simulink model "Test_sensor_drift"  (R2017b)
settings: Solver=VariableStepAuto  StartTime=0.0  StopTime=10.0  RelTol=1e-3
settings Model: Creator=dc0069  LastModifiedBy=dc0069

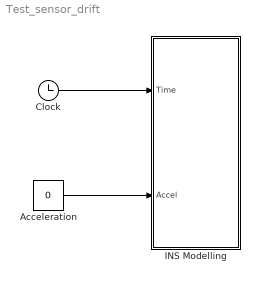
== system Test_sensor_drift ==
  Acceleration : Constant  Value=0
  Clock : Clock
  INS Modelling : Subsystem
  wires:
  Clock/1 -> INS Modelling/1(Time)
  Acceleration/1 -> INS Modelling/2(Accel)

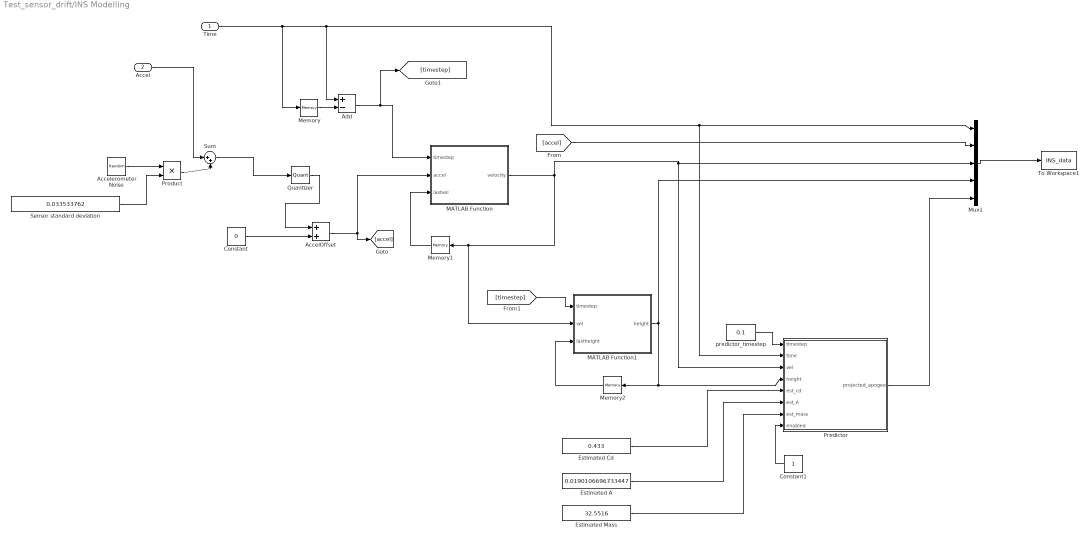
== system Test_sensor_drift/INS Modelling ==
  Time : Inport  SampleTime=.1
  Accel : Inport  Port=2  SampleTime=.1
  AccelOffset : Sum
  Accelerometer Noise : RandomNumber  Seed=3784  SampleTime=0.1  VectorParams1D=off
  Add : Sum  Inputs=+-
  Constant : Constant  Value=0
  Constant1 : Constant
  Estimated A : Constant  Value=0.0190106696733447
  Estimated Cd : Constant  Value=0.433
  Estimated Mass : Constant  Value=32.5516
  MATLAB Function : MATLAB Function  TreatAsAtomicUnit=on
  MATLAB Function1 : MATLAB Function  TreatAsAtomicUnit=on
  Memory : Memory
  Memory1 : Memory
  Memory2 : Memory
  Mux1 : Mux  Inputs=5
  Predictor : MATLAB Function  TreatAsAtomicUnit=on
  Product : Product
  Quantizer : Quantizer  QuantizationInterval=.01
  Sensor standard deviation : Constant  Value=0.033533762
  Sum : Sum  Inputs=|++
  To Workspace1 : ToWorkspace  VariableName=INS_data  SampleTime=.1
  "predictor_timestep " : Constant  Value=0.1
  wires:
  Accel/1 -> Sum/1
  Mux1/1 -> To Workspace1/1
  Time/1 -> Add/1, Predictor/2(time), Mux1/1, Memory/1
  AccelOffset/1 -> MATLAB Function/2(accel), [accel]
  Memory/1 -> Add/2
  Add/1 -> [timestep], MATLAB Function/1(timestep)
  [accel] -> Mux1/2
  MATLAB Function/1(velocity) -> MATLAB Function1/2(vel), Memory1/1, Mux1/3, Predictor/3(vel)
  Memory1/1 -> MATLAB Function/3(lastvel)
  Sum/1 -> Quantizer/1
  [timestep] -> MATLAB Function1/1(timestep)
  MATLAB Function1/1(height) -> Mux1/4, Predictor/4(height), Memory2/1
  Memory2/1 -> MATLAB Function1/3(lastheight)
  Predictor/1(projected_apogee) -> Mux1/5
  Quantizer/1 -> AccelOffset/1
  Constant/1 -> AccelOffset/2
  Estimated Cd/1 -> Predictor/5(est_cd)
  Estimated A/1 -> Predictor/6(est_A)
  Estimated Mass/1 -> Predictor/7(est_mass)
  "predictor_timestep "/1 -> Predictor/1(timestep)
  Sensor standard deviation/1 -> Product/2
  Accelerometer Noise/1 -> Product/1
  Product/1 -> Sum/2
  Constant1/1 -> Predictor/8(enabled)

== matlab function Test_sensor_drift/INS Modelling/MATLAB Function ==
  data: timestep input; accel input; lastvel input; velocity output
function velocity = fcn(timestep, accel, lastvel)
velocity = lastvel + timestep * accel;
end

== matlab function Test_sensor_drift/INS Modelling/MATLAB Function1 ==
  data: timestep input; vel input; lastheight input; height output
function height = fcn(timestep, vel, lastheight)

height = lastheight + timestep * vel;
end

== matlab function Test_sensor_drift/INS Modelling/Predictor ==
  data: timestep input; time input; projected_apogee output; vel input; height input; est_cd input; est_A input; est_mass input; enabled input
function projected_apogee = fcn(timestep, time, vel, height, est_cd, est_A, est_mass, enabled)
if (enabled == 1)
    max_time = 100; %In case something goes wrong it doesn't go into an infinite loop
    
    %cd = 0.433;
    %A = 0.0190106696733447;
    %mass = 32.5516;
    
    cd = est_cd;
    A = est_A;
    mass = est_mass;
    
    while(true)
        lastheight = height;
        time = time + timestep;
        
        p = getStandardPressure(height);
        rho = p/(287.058*(getStandardTemperature(getGeopotential(height/1000))));
        
        accel = -9.81 - ((1/2)*rho*A*cd*vel^2)/mass;
        vel = vel + accel*timestep;
        height = height + vel*timestep;
        
        if(lastheight > height || time > max_time); break; end
    end
end
projected_apogee = height;
end

% stuff below this stolen from wikipedia
function pressure = getStandardPressure( altitude)

altitude = altitude / 1000.0;
geopot_height = getGeopotential(altitude);

t = getStandardTemperature(geopot_height);

pressure = 0;
if (geopot_height <= 11)
    pressure = 101325 * (288.15 / t)^( -5.255877);
elseif (geopot_height <= 20)
    pressure = 22632.06 * exp(-0.1577 * (geopot_height - 11));
elseif (geopot_height <= 32)
    pressure = 5474.889 * (216.65 / t)^( 34.16319);
elseif (geopot_height <= 47)
    pressure = 868.0187 * (228.65 / t)^( 12.2011);
elseif (geopot_height <= 51)
    pressure = 110.9063 * exp(-0.1262 * (geopot_height - 47));
elseif (geopot_height <= 71)
    pressure = 66.93887 * (270.65 / t)^( -12.2011);
elseif (geopot_height <= 84.85)
    pressure = 3.956420 * (214.65 / t)^( -17.0816);
end

end

function temperature = getStandardTemperature(geopot_height)

temperature = 273.15;
if (geopot_height <= 11)
    temperature = 288.15 - (6.5 * geopot_height);
elseif (geopot_height <= 20)
    temperature = 216.65;
elseif (geopot_height <= 32)
    temperature = 196.65 + geopot_height;
elseif (geopot_height <= 47)
    temperature = 228.65 + 2.8 * (geopot_height - 32);
elseif (geopot_height <= 51)
    temperature = 270.65;
elseif (geopot_height <= 71)
    temperature = 270.65 - 2.8 * (geopot_height - 51);
elseif (geopot_height <= 84.85)
    temperature = 214.65 - 2 * (geopot_height - 71); 
end

end

function geopot = getGeopotential(altitude_km)

EARTH_RADIUS = 6356.766;

geopot = EARTH_RADIUS * altitude_km / (EARTH_RADIUS + altitude_km);
end
